simulink model "taskBasedWalking"  (Simulink 8.8)
settings: Solver=FixedStepDiscrete  StartTime=0.0  StopTime=Config.t_end  FixedStep=Config.t_step  RelTol=1e-3  EnableMultiTasking=on
InitFcn:
  | cd(fileparts(which(bdroot)));
  | initTaskBasedWalking;
StopFcn:
  | cd(fileparts(which(bdroot)));
  | stopTaskBasedWalking;
undefined symbols (not defined in the file or in its folder): biasVectorConstraint_feet, Config, ConstraintMatrix_feet, DiscIntNeverNeededParam, Gains, ROBOT_DOF, Sat
libraries: WBToolboxLibrary x78
(part 1 of 3)
settings Model: SuppressorTable=22 serialization::archive 11 0 6 0 0 0 11 0  Creator=gnava  LastModifiedBy=gabri
settings DataIOCC: LimitDataPoints=off  SaveFormat=Dataset  SignalLoggingSaveFormat=Dataset
settings OptimizationCC: LifeSpan=auto
settings DebuggingCC: UnderspecifiedInitializationDetection=Simplified  MergeDetectMultiDrivingBlocksExec=error  FcnCallInpInsideContextMsg=error  StateNameClashWarn=none  SFUnexpectedBacktrackingDiag=error  SFNoUnconditionalDefaultTransitionDiag=error
settings HardwareCC: ProdBitPerPointer=64  ProdBitPerSizeT=64  ProdBitPerPtrDiffT=64  ProdLargestAtomicFloat=Float  ProdIntDivRoundTo=Zero  ProdEndianess=LittleEndian  ProdWordSize=64  ProdHWDeviceType=Intel->x86-64 (Windows64)
settings ModelReferenceCC: PropagateSignalLabelsOutOfModel=on
settings GRTTargetCC: TargetLangStandard=C99 (ISO)  GeneratePreprocessorConditionals=Use local settings  CombineOutputUpdateFcns=on  GRTInterface=off
settings ConfigComp: CovSFcnEnable=off

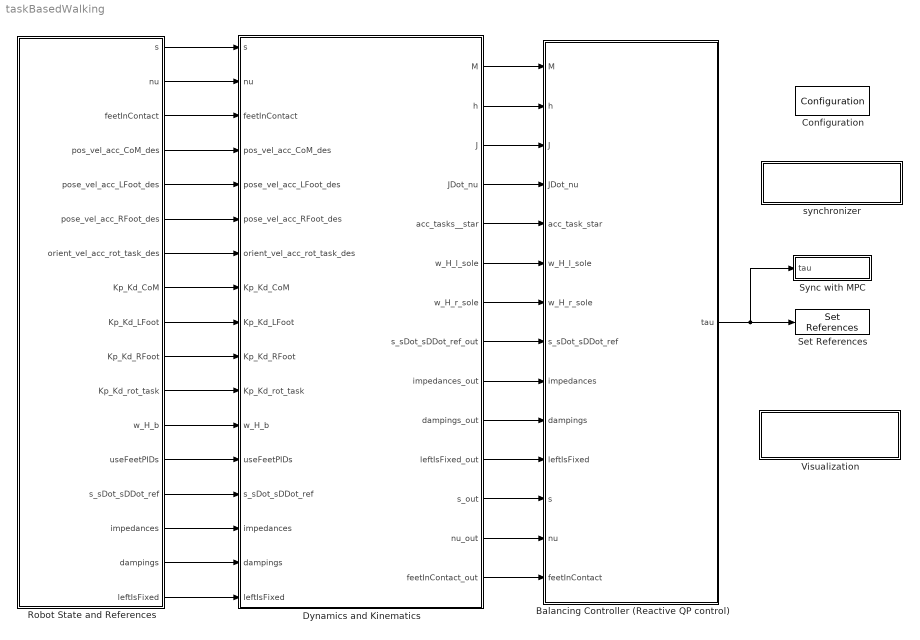
== system taskBasedWalking ==
  Balancing Controller (Reactive QP control) : Subsystem
  Configuration : WBToolboxLibrary/Utilities/Configuration  ConfigSource=Workspace  ConfigObject='WBTConfigRobot'  RobotName='icub'  UrdfFile='model.urdf'  ControlledJoints={'l_elbow','l_shoulder_pitch','torso_roll'}  ControlBoardsNames={'left_arm','right_arm','torso'}  LocalName='WBT'  GravityVector=[0,0,-9.81]
  Dynamics and Kinematics : Subsystem
  Robot State and References : Subsystem
  Set References : WBToolboxLibrary/wholeBodyActuators/Set References  controlType=Torque  refSpeed=50
  Sync with MPC : Subsystem
      mask Display: disp('Sync with MPC')
  Visualization : Subsystem
      mask Display: disp('VISUALIZE AND DUMP DATA')
  synchronizer : Subsystem
      mask Display: disp('SYNCHRONIZER')
  wires:
  Balancing Controller (Reactive QP control)/1(tau) -> Sync with MPC/1(tau), Set References/1
  Robot State and References/1(s) -> Dynamics and Kinematics/1(s)
  Robot State and References/2(nu) -> Dynamics and Kinematics/2(nu)
  Robot State and References/3(feetInContact) -> Dynamics and Kinematics/3(feetInContact)
  Robot State and References/4(pos_vel_acc_CoM_des) -> Dynamics and Kinematics/4(pos_vel_acc_CoM_des)
  Robot State and References/5(pose_vel_acc_LFoot_des) -> Dynamics and Kinematics/5(pose_vel_acc_LFoot_des)
  Robot State and References/6(pose_vel_acc_RFoot_des) -> Dynamics and Kinematics/6(pose_vel_acc_RFoot_des)
  Robot State and References/7(orient_vel_acc_rot_task_des) -> Dynamics and Kinematics/7(orient_vel_acc_rot_task_des)
  Robot State and References/8(Kp_Kd_CoM) -> Dynamics and Kinematics/8(Kp_Kd_CoM)
  Robot State and References/9(Kp_Kd_LFoot) -> Dynamics and Kinematics/9(Kp_Kd_LFoot)
  Robot State and References/10(Kp_Kd_RFoot) -> Dynamics and Kinematics/10(Kp_Kd_RFoot)
  Robot State and References/11(Kp_Kd_rot_task) -> Dynamics and Kinematics/11(Kp_Kd_rot_task)
  Robot State and References/12(w_H_b) -> Dynamics and Kinematics/12(w_H_b)
  Robot State and References/13("useFeetPIDs ") -> Dynamics and Kinematics/13(useFeetPIDs)
  Robot State and References/14(s_sDot_sDDot_ref) -> Dynamics and Kinematics/14(s_sDot_sDDot_ref)
  Robot State and References/15(impedances) -> Dynamics and Kinematics/15(impedances)
  Robot State and References/16(dampings) -> Dynamics and Kinematics/16(dampings)
  Robot State and References/17(leftIsFixed) -> Dynamics and Kinematics/17(leftIsFixed)
  Dynamics and Kinematics/1(M) -> Balancing Controller (Reactive QP control)/1(M)
  Dynamics and Kinematics/2(h) -> Balancing Controller (Reactive QP control)/2(h)
  Dynamics and Kinematics/3(J) -> Balancing Controller (Reactive QP control)/3(J)
  Dynamics and Kinematics/4(JDot_nu) -> Balancing Controller (Reactive QP control)/4(JDot_nu)
  Dynamics and Kinematics/5(acc_tasks__star) -> Balancing Controller (Reactive QP control)/5(acc_task_star)
  Dynamics and Kinematics/6(w_H_l_sole) -> Balancing Controller (Reactive QP control)/6(w_H_l_sole)
  Dynamics and Kinematics/7(w_H_r_sole) -> Balancing Controller (Reactive QP control)/7(w_H_r_sole)
  Dynamics and Kinematics/8(s_sDot_sDDot_ref_out) -> Balancing Controller (Reactive QP control)/8(s_sDot_sDDot_ref)
  Dynamics and Kinematics/9(impedances_out) -> Balancing Controller (Reactive QP control)/9(impedances)
  Dynamics and Kinematics/10(dampings_out) -> Balancing Controller (Reactive QP control)/10(dampings)
  Dynamics and Kinematics/11(leftIsFixed_out) -> Balancing Controller (Reactive QP control)/11(leftIsFixed)
  Dynamics and Kinematics/12(s_out) -> Balancing Controller (Reactive QP control)/12(s)
  Dynamics and Kinematics/13(nu_out) -> Balancing Controller (Reactive QP control)/13(nu)
  Dynamics and Kinematics/14(feetInContact_out) -> Balancing Controller (Reactive QP control)/14(feetInContact)

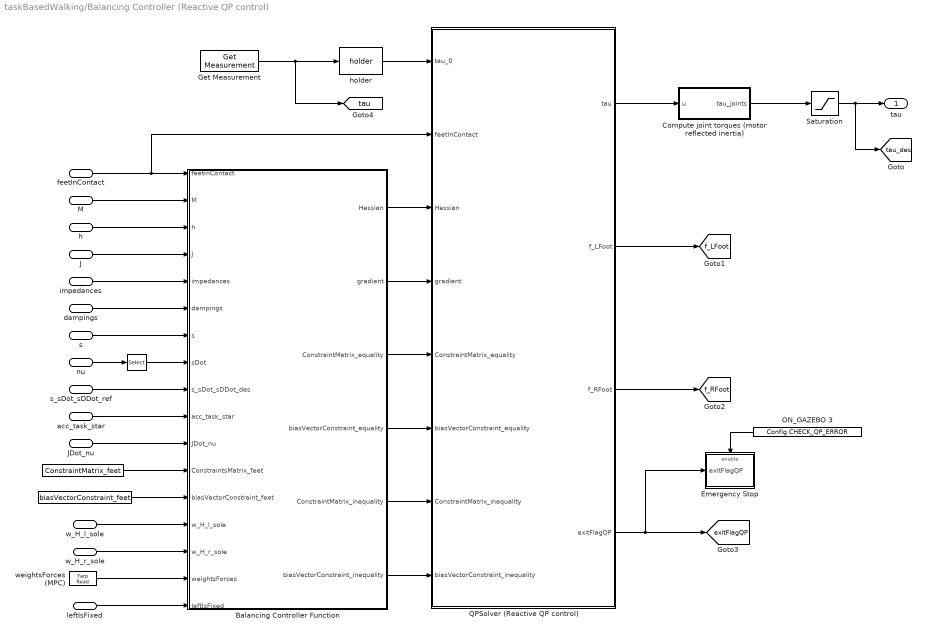
== system taskBasedWalking/Balancing Controller (Reactive QP control) ==
  M : Inport
  h : Inport  Port=2
  J : Inport  Port=3
  JDot_nu : Inport  Port=4
  acc_task_star : Inport  Port=5
  w_H_l_sole : Inport  Port=6
  w_H_r_sole : Inport  Port=7
  s_sDot_sDDot_ref : Inport  Port=8
  impedances : Inport  Port=9
  dampings : Inport  Port=10
  leftIsFixed : Inport  Port=11
  s : Inport  Port=12
  nu : Inport  Port=13
  feetInContact : Inport  Port=14
  "   " : Constant  Value=ConstraintMatrix_feet
  "      " : Constant  Value=biasVectorConstraint_feet
  "             " : Selector  InputPortWidth=ROBOT_DOF+6  IndexOptions=Index vector (dialog)  Indices=[7:ROBOT_DOF+6]  OutputSizes=1
  Balancing Controller Function : MATLAB Function  TreatAsAtomicUnit=on
  Compute joint torques (motor reflected inertia) : Subsystem
  Emergency Stop : Subsystem
  Get Measurement : WBToolboxLibrary/wholeBodyStates/Get Measurement  measuredType=Joints Torque
  ON_GAZEBO 3 : Constant  Value=Config.CHECK_QP_ERROR
  QPSolver (Reactive QP control) : Subsystem
  Saturation : Saturate  UpperLimit=Sat.tau_max  LowerLimit=-Sat.tau_max
  "holder " : WBToolboxLibrary/Utilities/holder 
  weightsForces (MPC) : WBToolboxLibrary/Utilities/Yarp Read  portName=Ports.FORCE_WEIGHTS  signalSize=2  timeout=0.5  blocking=off  timestamp=off  autoconnect=on  errorOnConnection=off
  tau : Outport
  tag scope: exitFlagQP=global, f_LFoot=global, f_RFoot=global, tau=global, tau_des=global
  wires:
  QPSolver (Reactive QP control)/1(tau) -> Compute joint torques (motor reflected inertia)/1(u)
  "holder "/1 -> QPSolver (Reactive QP control)/1(tau_0)
  Balancing Controller Function/3(ConstraintMatrix_equality) -> QPSolver (Reactive QP control)/5(ConstraintMatrix_equality)
  Balancing Controller Function/6(biasVectorConstraint_inequality) -> QPSolver (Reactive QP control)/8(biasVectorConstraint_inequality)
  Balancing Controller Function/2(gradient) -> QPSolver (Reactive QP control)/4(gradient)
  Balancing Controller Function/4(biasVectorConstraint_equality) -> QPSolver (Reactive QP control)/6(biasVectorConstraint_equality)
  Balancing Controller Function/5(ConstraintMatrix_inequality) -> QPSolver (Reactive QP control)/7(ConstraintMatrix_inequality)
  w_H_r_sole/1 -> Balancing Controller Function/15(w_H_r_sole)
  w_H_l_sole/1 -> Balancing Controller Function/14(w_H_l_sole)
  "      "/1 -> Balancing Controller Function/13(biasVectorConstraint_feet)
  "   "/1 -> Balancing Controller Function/12(ConstraintsMatrix_feet)
  JDot_nu/1 -> Balancing Controller Function/11(JDot_nu)
  acc_task_star/1 -> Balancing Controller Function/10(acc_task_star)
  s_sDot_sDDot_ref/1 -> Balancing Controller Function/9(s_sDot_sDDot_des)
  nu/1 -> "             "/1
  s/1 -> Balancing Controller Function/7(s)
  dampings/1 -> Balancing Controller Function/6(dampings)
  impedances/1 -> Balancing Controller Function/5(impedances)
  J/1 -> Balancing Controller Function/4(J)
  h/1 -> Balancing Controller Function/3(h)
  M/1 -> Balancing Controller Function/2(M)
  Get Measurement/1 -> [tau], "holder "/1
  "             "/1 -> Balancing Controller Function/8(sDot)
  Saturation/1 -> tau/1, [tau_des]
  Balancing Controller Function/1(Hessian) -> QPSolver (Reactive QP control)/3(Hessian)
  feetInContact/1 -> Balancing Controller Function/1(feetInContact), QPSolver (Reactive QP control)/2(feetInContact)
  QPSolver (Reactive QP control)/2(f_LFoot) -> [f_LFoot]
  QPSolver (Reactive QP control)/3(f_RFoot) -> [f_RFoot]
  QPSolver (Reactive QP control)/4(exitFlagQP) -> Emergency Stop/1(exitFlagQP), [exitFlagQP]
  ON_GAZEBO 3/1 -> Emergency Stop/Enable
  Compute joint torques (motor reflected inertia)/1(tau_joints) -> Saturation/1
  weightsForces (MPC)/1 -> Balancing Controller Function/16(weightsForces)
  leftIsFixed/1 -> Balancing Controller Function/17(leftIsFixed)

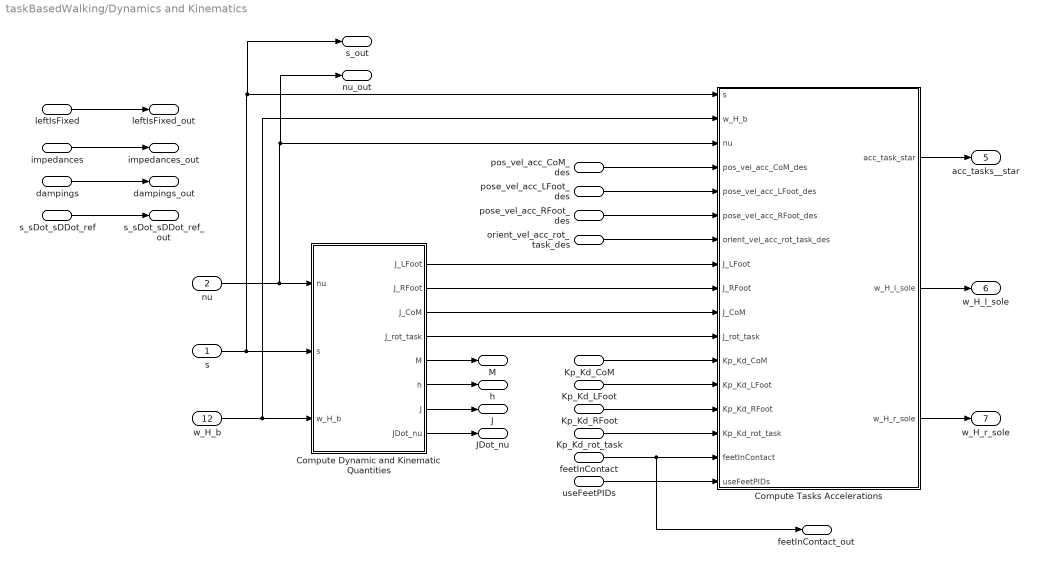
== system taskBasedWalking/Dynamics and Kinematics ==
  s : Inport
  nu : Inport  Port=2
  feetInContact : Inport  Port=3
  pos_vel_acc_CoM_des : Inport  Port=4
  pose_vel_acc_LFoot_des : Inport  Port=5
  pose_vel_acc_RFoot_des : Inport  Port=6
  orient_vel_acc_rot_task_des : Inport  Port=7
  Kp_Kd_CoM : Inport  Port=8
  Kp_Kd_LFoot : Inport  Port=9
  Kp_Kd_RFoot : Inport  Port=10
  Kp_Kd_rot_task : Inport  Port=11
  w_H_b : Inport  Port=12
  useFeetPIDs : Inport  Port=13
  s_sDot_sDDot_ref : Inport  Port=14
  impedances : Inport  Port=15
  dampings : Inport  Port=16
  leftIsFixed : Inport  Port=17
  Compute Dynamic and Kinematic Quantities : Subsystem
  Compute Tasks Accelerations : Subsystem
  M : Outport
  h : Outport  Port=2
  J : Outport  Port=3
  JDot_nu : Outport  Port=4
  acc_tasks__star : Outport  Port=5
  w_H_l_sole : Outport  Port=6
  w_H_r_sole : Outport  Port=7
  s_sDot_sDDot_ref_out : Outport  Port=8
  impedances_out : Outport  Port=9
  dampings_out : Outport  Port=10
  leftIsFixed_out : Outport  Port=11
  s_out : Outport  Port=12
  nu_out : Outport  Port=13
  feetInContact_out : Outport  Port=14
  wires:
  pos_vel_acc_CoM_des/1 -> Compute Tasks Accelerations/4(pos_vel_acc_CoM_des)
  pose_vel_acc_LFoot_des/1 -> Compute Tasks Accelerations/5(pose_vel_acc_LFoot_des)
  pose_vel_acc_RFoot_des/1 -> Compute Tasks Accelerations/6(pose_vel_acc_RFoot_des)
  orient_vel_acc_rot_task_des/1 -> Compute Tasks Accelerations/7(orient_vel_acc_rot_task_des)
  Kp_Kd_CoM/1 -> Compute Tasks Accelerations/12(Kp_Kd_CoM)
  Kp_Kd_LFoot/1 -> Compute Tasks Accelerations/13(Kp_Kd_LFoot)
  Kp_Kd_RFoot/1 -> Compute Tasks Accelerations/14(Kp_Kd_RFoot)
  Kp_Kd_rot_task/1 -> Compute Tasks Accelerations/15(Kp_Kd_rot_task)
  nu/1 -> Compute Dynamic and Kinematic Quantities/1(nu), nu_out/1, Compute Tasks Accelerations/3(nu)
  s/1 -> Compute Dynamic and Kinematic Quantities/2(s), s_out/1, Compute Tasks Accelerations/1(s)
  w_H_b/1 -> Compute Dynamic and Kinematic Quantities/3(w_H_b), Compute Tasks Accelerations/2(w_H_b)
  Compute Dynamic and Kinematic Quantities/6(h) -> h/1
  Compute Dynamic and Kinematic Quantities/1(J_LFoot) -> Compute Tasks Accelerations/8(J_LFoot)
  Compute Dynamic and Kinematic Quantities/2(J_RFoot) -> Compute Tasks Accelerations/9(J_RFoot)
  Compute Dynamic and Kinematic Quantities/3(J_CoM) -> Compute Tasks Accelerations/10(J_CoM)
  Compute Dynamic and Kinematic Quantities/5(M) -> M/1
  Compute Dynamic and Kinematic Quantities/4(J_rot_task) -> Compute Tasks Accelerations/11(J_rot_task)
  Compute Dynamic and Kinematic Quantities/7(J) -> J/1
  Compute Dynamic and Kinematic Quantities/8(JDot_nu) -> JDot_nu/1
  Compute Tasks Accelerations/2(w_H_l_sole) -> w_H_l_sole/1
  Compute Tasks Accelerations/3(w_H_r_sole) -> w_H_r_sole/1
  Compute Tasks Accelerations/1(acc_task_star) -> acc_tasks__star/1
  useFeetPIDs/1 -> Compute Tasks Accelerations/17(useFeetPIDs)
  leftIsFixed/1 -> leftIsFixed_out/1
  impedances/1 -> impedances_out/1
  dampings/1 -> dampings_out/1
  s_sDot_sDDot_ref/1 -> s_sDot_sDDot_ref_out/1
  feetInContact/1 -> feetInContact_out/1, Compute Tasks Accelerations/16(feetInContact)

== system taskBasedWalking/Robot State and References ==
  Gain Scheduling : Subsystem
  ON_GAZEBO 1 : Constant  Value=Config.CHECK_LIMITS
  "Smooth References " : Subsystem
  State Machine : Subsystem
  emergency stop: joint limits : Subsystem
  s : Outport
  nu : Outport  Port=2
  feetInContact : Outport  Port=3
  pos_vel_acc_CoM_des : Outport  Port=4
  pose_vel_acc_LFoot_des : Outport  Port=5
  pose_vel_acc_RFoot_des : Outport  Port=6
  orient_vel_acc_rot_task_des : Outport  Port=7
  Kp_Kd_CoM : Outport  Port=8
  Kp_Kd_LFoot : Outport  Port=9
  Kp_Kd_RFoot : Outport  Port=10
  Kp_Kd_rot_task : Outport  Port=11
  w_H_b : Outport  Port=12
  "useFeetPIDs " : Outport  Port=13
  s_sDot_sDDot_ref : Outport  Port=14
  impedances : Outport  Port=15
  dampings : Outport  Port=16
  leftIsFixed : Outport  Port=17
  wires:
  Gain Scheduling/1(Kp_Kd_CoM) -> Kp_Kd_CoM/1
  Gain Scheduling/2(Kp_Kd_LFoot) -> Kp_Kd_LFoot/1
  Gain Scheduling/3(Kp_Kd_RFoot) -> Kp_Kd_RFoot/1
  Gain Scheduling/4(Kp_Kd_rot_task) -> Kp_Kd_rot_task/1
  Gain Scheduling/5(impedances) -> impedances/1
  Gain Scheduling/6(dampings) -> dampings/1
  "Smooth References "/1(pos_vel_acc_CoM_des) -> pos_vel_acc_CoM_des/1
  "Smooth References "/2(pose_vel_acc_LFoot_des) -> pose_vel_acc_LFoot_des/1
  "Smooth References "/3(pose_vel_acc_RFoot_des) -> pose_vel_acc_RFoot_des/1
  "Smooth References "/4(orient_vel_acc_rot_task_des) -> orient_vel_acc_rot_task_des/1
  "Smooth References "/5(s_sDot_sDDot_ref) -> s_sDot_sDDot_ref/1
  ON_GAZEBO 1/1 -> emergency stop: joint limits/Enable
  State Machine/1(s) -> s/1, emergency stop: joint limits/1(s   EMERGENCY STOP)
  State Machine/2(w_H_b) -> w_H_b/1
  State Machine/3(nu) -> nu/1
  State Machine/4(feetInContact) -> feetInContact/1
  State Machine/5(leftIsFixed) -> leftIsFixed/1
  State Machine/7(state) -> "Smooth References "/1(state), Gain Scheduling/1(state)
  State Machine/8(references_CoM) -> "Smooth References "/2(references_CoM)
  State Machine/9(references_LFoot) -> "Smooth References "/3(references_LFoot)
  State Machine/10(references_RFoot) -> "Smooth References "/4(references_RFoot)
  State Machine/11(references_rot_task) -> "Smooth References "/5(references_rot_task)
  State Machine/12(references_s) -> "Smooth References "/6(references_s)
  State Machine/6(useFeetPIDs) -> "useFeetPIDs "/1

== system taskBasedWalking/Sync with MPC ==
  tau : Inport
  Clock : Clock
  Gain : Gain  Gain=0
  Mux : Mux  Inputs=2
  Selector : Selector  InputPortWidth=ROBOT_DOF  IndexOptions=Index vector (dialog)  Indices=[1]  OutputSizes=1
  Yarp Write : WBToolboxLibrary/Utilities/Yarp Write  portName=Ports.ACK  autoconnect=on  errorOnConnection=off
  wires:
  Clock/1 -> Mux/2
  tau/1 -> Selector/1
  Mux/1 -> Yarp Write/1
  Selector/1 -> Gain/1
  Gain/1 -> Mux/1

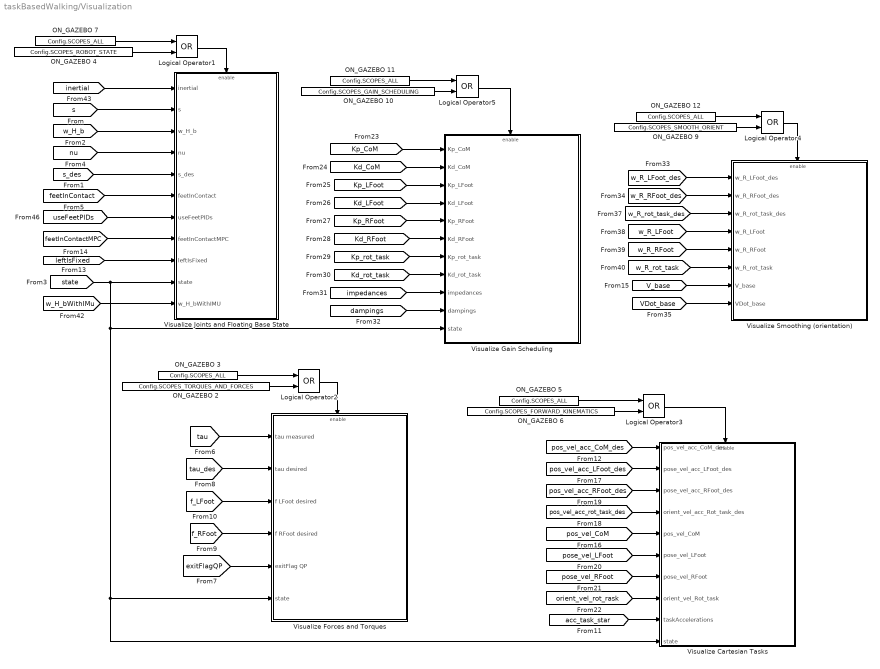
== system taskBasedWalking/Visualization ==
  Logical Operator{1..5} (5 alike) : Logic  Operator=OR  AllPortsSameDT=off  OutDataTypeStr=boolean
  ON_GAZEBO 10 : Constant  Value=Config.SCOPES_GAIN_SCHEDULING
  ON_GAZEBO {3,5,7,11..12} (5 alike) : Constant  Value=Config.SCOPES_ALL
  ON_GAZEBO 2 : Constant  Value=Config.SCOPES_TORQUES_AND_FORCES
  ON_GAZEBO 4 : Constant  Value=Config.SCOPES_ROBOT_STATE
  ON_GAZEBO 6 : Constant  Value=Config.SCOPES_FORWARD_KINEMATICS
  ON_GAZEBO 9 : Constant  Value=Config.SCOPES_SMOOTH_ORIENT
  Visualize Cartesian Tasks : Subsystem
  Visualize Forces and Torques : Subsystem
  Visualize Gain Scheduling : Subsystem
  Visualize Joints and Floating Base State : Subsystem
  Visualize Smoothing (orientation) : Subsystem
  wires:
  [s] -> Visualize Joints and Floating Base State/2(s)
  [w_H_b] -> Visualize Joints and Floating Base State/3(w_H_b)
  [s_des] -> Visualize Joints and Floating Base State/5(s_des)
  [nu] -> Visualize Joints and Floating Base State/4(nu)
  [state] -> Visualize Cartesian Tasks/10(state), Visualize Forces and Torques/6(state), Visualize Gain Scheduling/11(state), Visualize Joints and Floating Base State/10(state)
  [tau] -> Visualize Forces and Torques/1(tau measured)
  [tau_des] -> Visualize Forces and Torques/2(tau desired)
  [f_LFoot] -> Visualize Forces and Torques/3(f LFoot desired)
  [f_RFoot] -> Visualize Forces and Torques/4(f RFoot desired)
  [exitFlagQP] -> Visualize Forces and Torques/5(exitFlag QP)
  ON_GAZEBO 4/1 -> Logical Operator1/2
  ON_GAZEBO 7/1 -> Logical Operator1/1
  Logical Operator1/1 -> Visualize Joints and Floating Base State/Enable
  [feetInContact] -> Visualize Joints and Floating Base State/6(feetInContact)
  Logical Operator2/1 -> Visualize Forces and Torques/Enable
  ON_GAZEBO 3/1 -> Logical Operator2/1
  ON_GAZEBO 2/1 -> Logical Operator2/2
  ON_GAZEBO 6/1 -> Logical Operator3/2
  Logical Operator3/1 -> Visualize Cartesian Tasks/Enable
  ON_GAZEBO 5/1 -> Logical Operator3/1
  [pos_vel_acc_CoM_des] -> Visualize Cartesian Tasks/1(pos_vel_acc_CoM_des)
  [pos_vel_acc_LFoot_des] -> Visualize Cartesian Tasks/2(pose_vel_acc_LFoot_des)
  [pos_vel_acc_RFoot_des] -> Visualize Cartesian Tasks/3(pose_vel_acc_RFoot_des)
  [pos_vel_acc_rot_task_des] -> Visualize Cartesian Tasks/4(orient_vel_acc_Rot_task_des)
  [pos_vel_CoM] -> Visualize Cartesian Tasks/5(pos_vel_CoM)
  [pose_vel_LFoot] -> Visualize Cartesian Tasks/6(pose_vel_LFoot)
  [pose_vel_RFoot] -> Visualize Cartesian Tasks/7(pose_vel_RFoot)
  [orient_vel_rot_rask] -> Visualize Cartesian Tasks/8(orient_vel_Rot_task)
  ON_GAZEBO 10/1 -> Logical Operator5/2
  ON_GAZEBO 11/1 -> Logical Operator5/1
  Logical Operator5/1 -> Visualize Gain Scheduling/Enable
  [Kp_CoM] -> Visualize Gain Scheduling/1(Kp_CoM)
  [Kd_CoM] -> Visualize Gain Scheduling/2(Kd_CoM)
  [Kp_LFoot] -> Visualize Gain Scheduling/3(Kp_LFoot)
  [Kd_LFoot] -> Visualize Gain Scheduling/4(Kd_LFoot)
  [Kp_RFoot] -> Visualize Gain Scheduling/5(Kp_RFoot)
  [Kd_RFoot] -> Visualize Gain Scheduling/6(Kd_RFoot)
  [Kp_rot_task] -> Visualize Gain Scheduling/7(Kp_rot_task)
  [Kd_rot_task] -> Visualize Gain Scheduling/8(Kd_rot_task)
  [impedances] -> Visualize Gain Scheduling/9(impedances)
  [dampings] -> Visualize Gain Scheduling/10(dampings)
  ON_GAZEBO 9/1 -> Logical Operator4/2
  ON_GAZEBO 12/1 -> Logical Operator4/1
  Logical Operator4/1 -> Visualize Smoothing (orientation)/Enable
  [w_R_LFoot_des] -> Visualize Smoothing (orientation)/1(w_R_LFoot_des)
  [w_R_RFoot_des] -> Visualize Smoothing (orientation)/2(w_R_RFoot_des)
  [w_R_rot_task_des] -> Visualize Smoothing (orientation)/3(w_R_rot_task_des)
  [w_R_LFoot] -> Visualize Smoothing (orientation)/4(w_R_LFoot)
  [w_R_RFoot] -> Visualize Smoothing (orientation)/5(w_R_RFoot)
  [w_R_rot_task] -> Visualize Smoothing (orientation)/6(w_R_rot_task)
  [acc_task_star] -> Visualize Cartesian Tasks/9(taskAccelerations)
  [leftIsFixed] -> Visualize Joints and Floating Base State/9(leftIsFixed)
  [useFeetPIDs] -> Visualize Joints and Floating Base State/7(useFeetPIDs)
  [feetInContactMPC] -> Visualize Joints and Floating Base State/8(feetInContactMPC)
  [V_base] -> Visualize Smoothing (orientation)/7(V_base)
  [VDot_base] -> Visualize Smoothing (orientation)/8(VDot_base)
  [w_H_bWithIMu] -> Visualize Joints and Floating Base State/11(w_H_bWithIMU)
  [inertial] -> Visualize Joints and Floating Base State/1(inertial)

== system taskBasedWalking/synchronizer ==
  GAZEBO_SYNCHRONIZER : Subsystem
  Logical Operator : Logic  Operator=NOT  AllPortsSameDT=off  OutDataTypeStr=boolean
  "ON_GAZEBO " : Constant  Value=Config.ON_GAZEBO
  REAL_TIME_SYNC : Subsystem
  wires:
  Logical Operator/1 -> REAL_TIME_SYNC/Enable
  "ON_GAZEBO "/1 -> Logical Operator/1, GAZEBO_SYNCHRONIZER/Enable

== system taskBasedWalking/Balancing Controller (Reactive QP control)/Compute joint torques (motor reflected inertia) ==
  u : Inport
  " " : Constant  Value=Config.USE_MOTOR_REFLECTED_INERTIA
  "(transpose(T*Gamma))^{-1}*I_m*(T*Gamma)^{-1}" : MATLAB Function  TreatAsAtomicUnit=on
  Add : Sum  Inputs=-+
  DoFs converter1 : WBToolboxLibrary/Utilities/DoFs converter  yarp2WBIOption=From YARP to WBI
  DoFs converter2 : WBToolboxLibrary/Utilities/DoFs converter  yarp2WBIOption=From YARP to WBI
  Gain : Gain  Gain=Config.K_ff
  Get Measurement : WBToolboxLibrary/wholeBodyStates/Get Measurement  measuredType=Joints Acceleration
  Product : Product  Multiplication=Matrix(*)
  Switch : Switch  Criteria=u2 > Threshold
  joint accelerations : Scope  NumInputPorts=6
  motor reflected inertia ff terms : Scope  NumInputPorts=6
  tau_joints : Outport
  wires:
  Gain/1 -> Add/1
  Add/1 -> Switch/1
  " "/1 -> Switch/2
  Switch/1 -> tau_joints/1
  u/1 -> Add/2, Switch/3
  "(transpose(T*Gamma))^{-1}*I_m*(T*Gamma)^{-1}"/1(reflectedInertia) -> Product/1
  Get Measurement/1 -> DoFs converter1/1, Product/2
  DoFs converter1/4 -> joint accelerations/4  "left_leg"
  DoFs converter1/3 -> joint accelerations/3  "right_arm"
  DoFs converter1/5 -> joint accelerations/5  "right_leg"
  DoFs converter1/2 -> joint accelerations/2  "left_arm"
  DoFs converter1/1 -> joint accelerations/1  "torso"
  DoFs converter2/1 -> motor reflected inertia ff terms/1  "torso"
  DoFs converter2/3 -> motor reflected inertia ff terms/3  "right_arm"
  DoFs converter2/2 -> motor reflected inertia ff terms/2  "left_arm"
  DoFs converter2/5 -> motor reflected inertia ff terms/5  "right_leg"
  Product/1 -> DoFs converter2/1, Gain/1
  DoFs converter2/4 -> motor reflected inertia ff terms/4  "left_leg"

== system taskBasedWalking/Balancing Controller (Reactive QP control)/Emergency Stop ==
  exitFlagQP : Inport
  Enable : EnablePort
  Constant : Constant  Value=2
  Constant1 : Constant  Value=0  OutDataTypeStr=boolean
  Constant2 : Constant  OutDataTypeStr=boolean
  Stop Simulation : Stop
  Sum : Sum  Inputs=|++
  Switch : Switch  Criteria=u2 > Threshold  Threshold=0.1
  wires:
  exitFlagQP/1 -> Sum/1
  Sum/1 -> Switch/2
  Switch/1 -> Stop Simulation/1
  Constant/1 -> Sum/2
  Constant1/1 -> Switch/1
  Constant2/1 -> Switch/3

== system taskBasedWalking/Balancing Controller (Reactive QP control)/QPSolver (Reactive QP control) ==
  tau_0 : Inport
  feetInContact : Inport  Port=2
  Hessian : Inport  Port=3
  gradient : Inport  Port=4
  ConstraintMatrix_equality : Inport  Port=5
  biasVectorConstraint_equality : Inport  Port=6
  ConstraintMatrix_inequality : Inport  Port=7
  biasVectorConstraint_inequality : Inport  Port=8
  QPSolver : M-S-Function  FunctionName=QPBalancingMPC  Parameters=ROBOT_DOF, Sat, Config
  tau : Outport
  f_LFoot : Outport  Port=2
  f_RFoot : Outport  Port=3
  exitFlagQP : Outport  Port=4
  wires:
  gradient/1 -> QPSolver/4
  Hessian/1 -> QPSolver/3
  biasVectorConstraint_inequality/1 -> QPSolver/8
  feetInContact/1 -> QPSolver/2
  QPSolver/2 -> f_LFoot/1
  ConstraintMatrix_inequality/1 -> QPSolver/7
  biasVectorConstraint_equality/1 -> QPSolver/6
  ConstraintMatrix_equality/1 -> QPSolver/5
  tau_0/1 -> QPSolver/1
  QPSolver/1 -> tau/1
  QPSolver/3 -> f_RFoot/1
  QPSolver/4 -> exitFlagQP/1

== system taskBasedWalking/Dynamics and Kinematics/Compute Dynamic and Kinematic Quantities ==
  nu : Inport
  s : Inport  Port=2
  w_H_b : Inport  Port=3
  "  " : Selector  NumberOfDimensions=2  InputPortWidth=ROBOT_DOF+16  IndexOptions=Index vector (dialog),Index vector (dialog)  Indices=[1:3],[1:ROBOT_DOF+6]  OutputSizes=1,1
  "   " : Selector  InputPortWidth=6  IndexOptions=Index vector (dialog)  Indices=[1:3]  OutputSizes=1
  "     " : Selector  NumberOfDimensions=2  InputPortWidth=ROBOT_DOF+16  IndexOptions=Index vector (dialog),Index vector (dialog)  Indices=[4:6],[1:ROBOT_DOF+6]  OutputSizes=1,1
  "               " : Selector  InputPortWidth=6  IndexOptions=Index vector (dialog)  Indices=[4:6]  OutputSizes=1
  Jacobians and JDot_nu : Subsystem
  Mass Matrix and Bias Forces : Subsystem
  Matrix Concatenate : Concatenate  NumInputs=4  Mode=Multidimensional array
  Selector : Selector  InputPortWidth=ROBOT_DOF+6  IndexOptions=Index vector (dialog)  Indices=[1:6]  OutputSizes=1
  Selector1 : Selector  InputPortWidth=ROBOT_DOF+6  IndexOptions=Index vector (dialog)  Indices=[7:ROBOT_DOF+6]  OutputSizes=1
  Vector Concatenate : Concatenate  NumInputs=4
  J_LFoot : Outport
  J_RFoot : Outport  Port=2
  J_CoM : Outport  Port=3
  J_rot_task : Outport  Port=4
  M : Outport  Port=5
  h : Outport  Port=6
  J : Outport  Port=7
  JDot_nu : Outport  Port=8
  wires:
  "               "/1 -> Vector Concatenate/4
  "  "/1 -> J_CoM/1, Matrix Concatenate/3
  "     "/1 -> J_rot_task/1, Matrix Concatenate/4
  Vector Concatenate/1 -> JDot_nu/1
  Selector1/1 -> Mass Matrix and Bias Forces/3(sDot), Jacobians and JDot_nu/3(sDot)
  Matrix Concatenate/1 -> J/1
  nu/1 -> Selector/1, Selector1/1
  Selector/1 -> Mass Matrix and Bias Forces/2(nu_b), Jacobians and JDot_nu/2(nu_b)
  "   "/1 -> Vector Concatenate/3
  Mass Matrix and Bias Forces/2(M(q)) -> M/1
  Mass Matrix and Bias Forces/1(h(q,nu)) -> h/1
  s/1 -> Jacobians and JDot_nu/1(s), Mass Matrix and Bias Forces/1(s)
  w_H_b/1 -> Jacobians and JDot_nu/4(w_H_b), Mass Matrix and Bias Forces/4(w_H_b)
  Jacobians and JDot_nu/2(J_RFoot) -> J_RFoot/1, Matrix Concatenate/2
  Jacobians and JDot_nu/1(J_LFoot) -> J_LFoot/1, Matrix Concatenate/1
  Jacobians and JDot_nu/3(J_CoM) -> "  "/1
  Jacobians and JDot_nu/4(J_rot_task) -> "     "/1
  Jacobians and JDot_nu/5(JDot_nu_LFoot) -> Vector Concatenate/1
  Jacobians and JDot_nu/6(JDot_nu_RFoot) -> Vector Concatenate/2
  Jacobians and JDot_nu/7(JDot_nu_CoM) -> "   "/1
  Jacobians and JDot_nu/8(JDot_nu_rot_task) -> "               "/1

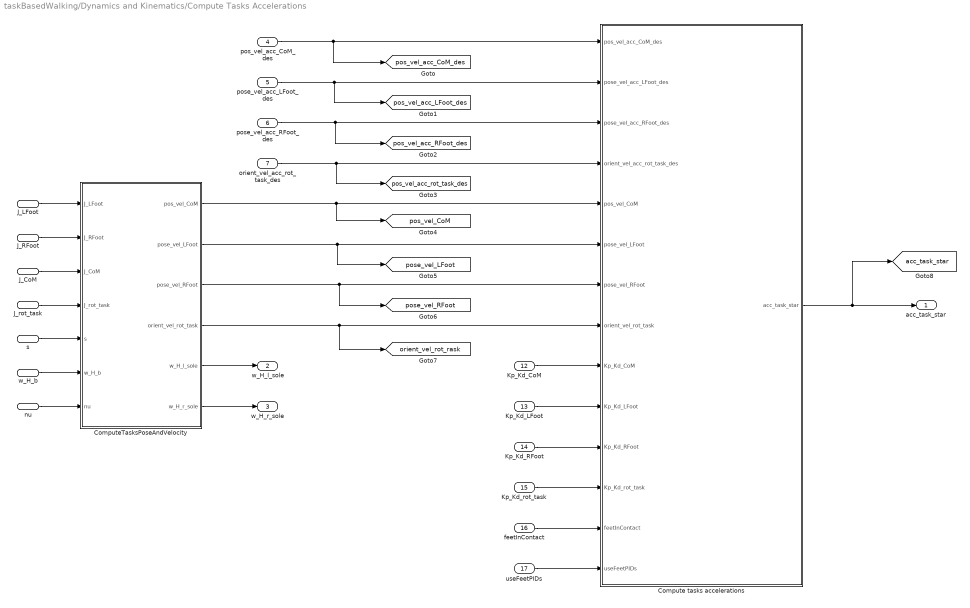
== system taskBasedWalking/Dynamics and Kinematics/Compute Tasks Accelerations ==
  s : Inport
  w_H_b : Inport  Port=2
  nu : Inport  Port=3
  pos_vel_acc_CoM_des : Inport  Port=4
  pose_vel_acc_LFoot_des : Inport  Port=5
  pose_vel_acc_RFoot_des : Inport  Port=6
  orient_vel_acc_rot_task_des : Inport  Port=7
  J_LFoot : Inport  Port=8
  J_RFoot : Inport  Port=9
  J_CoM : Inport  Port=10
  J_rot_task : Inport  Port=11
  Kp_Kd_CoM : Inport  Port=12
  Kp_Kd_LFoot : Inport  Port=13
  Kp_Kd_RFoot : Inport  Port=14
  Kp_Kd_rot_task : Inport  Port=15
  feetInContact : Inport  Port=16
  useFeetPIDs : Inport  Port=17
  Compute tasks accelerations : MATLAB Function  TreatAsAtomicUnit=on
  ComputeTasksPoseAndVelocity : Subsystem
  acc_task_star : Outport
  w_H_l_sole : Outport  Port=2
  w_H_r_sole : Outport  Port=3
  tag scope: acc_task_star=global, orient_vel_rot_rask=global, pos_vel_CoM=global, pos_vel_acc_CoM_des=global, pos_vel_acc_LFoot_des=global, pos_vel_acc_RFoot_des=global, pos_vel_acc_rot_task_des=global, pose_vel_LFoot=global, pose_vel_RFoot=global
  wires:
  pos_vel_acc_CoM_des/1 -> Compute tasks accelerations/1(pos_vel_acc_CoM_des), [pos_vel_acc_CoM_des]
  Kp_Kd_RFoot/1 -> Compute tasks accelerations/11(Kp_Kd_RFoot)
  Kp_Kd_rot_task/1 -> Compute tasks accelerations/12(Kp_Kd_rot_task)
  feetInContact/1 -> Compute tasks accelerations/13(feetInContact)
  pose_vel_acc_RFoot_des/1 -> [pos_vel_acc_RFoot_des], Compute tasks accelerations/3(pose_vel_acc_RFoot_des)
  Kp_Kd_LFoot/1 -> Compute tasks accelerations/10(Kp_Kd_LFoot)
  Kp_Kd_CoM/1 -> Compute tasks accelerations/9(Kp_Kd_CoM)
  orient_vel_acc_rot_task_des/1 -> [pos_vel_acc_rot_task_des], Compute tasks accelerations/4(orient_vel_acc_rot_task_des)
  pose_vel_acc_LFoot_des/1 -> [pos_vel_acc_LFoot_des], Compute tasks accelerations/2(pose_vel_acc_LFoot_des)
  Compute tasks accelerations/1(acc_task_star) -> [acc_task_star], acc_task_star/1
  ComputeTasksPoseAndVelocity/1(pos_vel_CoM) -> [pos_vel_CoM], Compute tasks accelerations/5(pos_vel_CoM)
  ComputeTasksPoseAndVelocity/4(orient_vel_rot_task) -> [orient_vel_rot_rask], Compute tasks accelerations/8(orient_vel_rot_task)
  J_LFoot/1 -> ComputeTasksPoseAndVelocity/1(J_LFoot)
  J_RFoot/1 -> ComputeTasksPoseAndVelocity/2(J_RFoot)
  J_CoM/1 -> ComputeTasksPoseAndVelocity/3(J_CoM)
  J_rot_task/1 -> ComputeTasksPoseAndVelocity/4(J_rot_task)
  s/1 -> ComputeTasksPoseAndVelocity/5(s)
  w_H_b/1 -> ComputeTasksPoseAndVelocity/6(w_H_b)
  nu/1 -> ComputeTasksPoseAndVelocity/7(nu)
  ComputeTasksPoseAndVelocity/2(pose_vel_LFoot) -> [pose_vel_LFoot], Compute tasks accelerations/6(pose_vel_LFoot)
  ComputeTasksPoseAndVelocity/3(pose_vel_RFoot) -> [pose_vel_RFoot], Compute tasks accelerations/7(pose_vel_RFoot)
  ComputeTasksPoseAndVelocity/5(w_H_l_sole) -> w_H_l_sole/1
  ComputeTasksPoseAndVelocity/6(w_H_r_sole) -> w_H_r_sole/1
  useFeetPIDs/1 -> Compute tasks accelerations/14(useFeetPIDs)

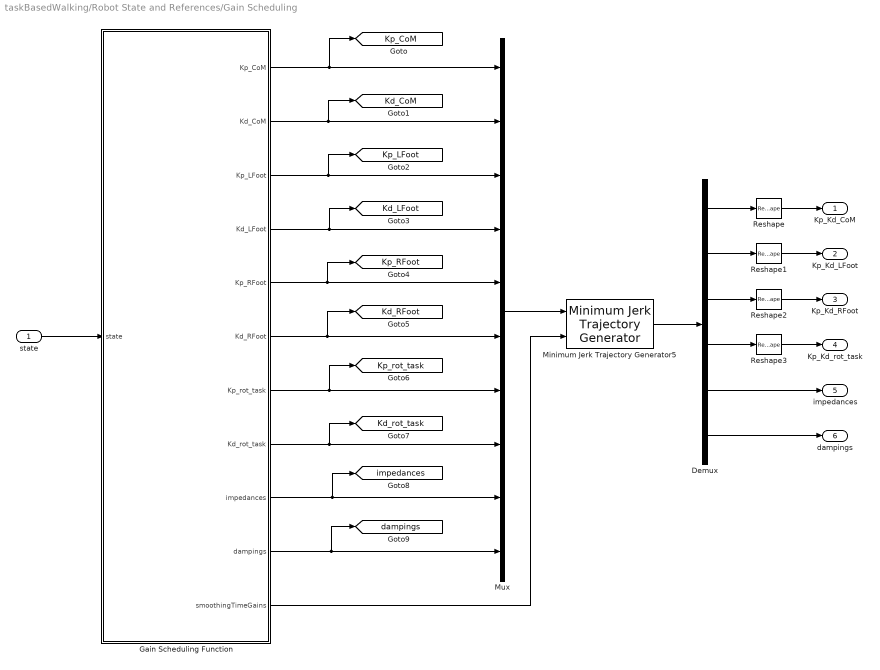
== system taskBasedWalking/Robot State and References/Gain Scheduling ==
  state : Inport
  Demux : Demux  Outputs=[6;12;12;6;ROBOT_DOF;ROBOT_DOF]
  Gain Scheduling Function : MATLAB Function  TreatAsAtomicUnit=on
  Minimum Jerk Trajectory Generator5 : WBToolboxLibrary/Utilities/Minimum Jerk Trajectory Generator  externalSettlingTime=on  settlingTime=3  sampleTime=Config.t_step  resetOnSettlingTime=off  firstDerivatives=off  secondDerivatives=off  explicitInitialValue=off
  Mux : Mux  Inputs=10
  Reshape : Reshape  OutputDimensionality=Customize  OutputDimensions=[3;2]
  Reshape1 : Reshape  OutputDimensionality=Customize  OutputDimensions=[6;2]
  Reshape2 : Reshape  OutputDimensionality=Customize  OutputDimensions=[6;2]
  Reshape3 : Reshape  OutputDimensionality=Customize  OutputDimensions=[3;2]
  Kp_Kd_CoM : Outport
  Kp_Kd_LFoot : Outport  Port=2
  Kp_Kd_RFoot : Outport  Port=3
  Kp_Kd_rot_task : Outport  Port=4
  impedances : Outport  Port=5
  dampings : Outport  Port=6
  tag scope: Kd_CoM=global, Kd_LFoot=global, Kd_RFoot=global, Kd_rot_task=global, Kp_CoM=global, Kp_LFoot=global, Kp_RFoot=global, Kp_rot_task=global, dampings=global, impedances=global
  wires:
  state/1 -> Gain Scheduling Function/1(state)
  Gain Scheduling Function/1(Kp_CoM) -> [Kp_CoM], Mux/1
  Gain Scheduling Function/2(Kd_CoM) -> [Kd_CoM], Mux/2
  Gain Scheduling Function/3(Kp_LFoot) -> [Kp_LFoot], Mux/3
  Gain Scheduling Function/4(Kd_LFoot) -> [Kd_LFoot], Mux/4
  Gain Scheduling Function/5(Kp_RFoot) -> [Kp_RFoot], Mux/5
  Gain Scheduling Function/6(Kd_RFoot) -> [Kd_RFoot], Mux/6
  Gain Scheduling Function/7(Kp_rot_task) -> [Kp_rot_task], Mux/7
  Gain Scheduling Function/8(Kd_rot_task) -> [Kd_rot_task], Mux/8
  Mux/1 -> Minimum Jerk Trajectory Generator5/1
  Gain Scheduling Function/9(impedances) -> [impedances], Mux/9
  Gain Scheduling Function/10(dampings) -> [dampings], Mux/10
  Gain Scheduling Function/11(smoothingTimeGains) -> Minimum Jerk Trajectory Generator5/2
  Minimum Jerk Trajectory Generator5/1 -> Demux/1
  Demux/1 -> Reshape/1
  Demux/2 -> Reshape1/1
  Demux/3 -> Reshape2/1
  Demux/4 -> Reshape3/1
  Reshape/1 -> Kp_Kd_CoM/1
  Reshape1/1 -> Kp_Kd_LFoot/1
  Reshape2/1 -> Kp_Kd_RFoot/1
  Reshape3/1 -> Kp_Kd_rot_task/1
  Demux/5 -> impedances/1
  Demux/6 -> dampings/1

== system taskBasedWalking/Robot State and References/Smooth References  ==
  state : Inport
  references_CoM : Inport  Port=2
  references_LFoot : Inport  Port=3
  references_RFoot : Inport  Port=4
  references_rot_task : Inport  Port=5
  references_s : Inport  Port=6
  Choose Smoothed or Direct References : Subsystem
  Selector1 : Selector  NumberOfDimensions=2  InputPortWidth=3  IndexOptions=Index vector (dialog),Index vector (dialog)  Indices=[1:3],1  OutputSizes=1,1
  Selector2 : Selector  NumberOfDimensions=2  InputPortWidth=3  IndexOptions=Index vector (dialog),Index vector (dialog)  Indices=[1:3],1  OutputSizes=1,1
  Selector3 : Selector  NumberOfDimensions=2  InputPortWidth=ROBOT_DOF  IndexOptions=Index vector (dialog),Index vector (dialog)  Indices=[1:ROBOT_DOF],1  OutputSizes=1,1
  Selector4 : Selector  NumberOfDimensions=2  InputPortWidth=3  IndexOptions=Index vector (dialog),Index vector (dialog)  Indices=[1:3],[1:3]  OutputSizes=1,1
  Selector6 : Selector  NumberOfDimensions=2  InputPortWidth=3  IndexOptions=Index vector (dialog),Index vector (dialog)  Indices=[1:3],1  OutputSizes=1,1
  Selector7 : Selector  NumberOfDimensions=2  InputPortWidth=ROBOT_DOF  IndexOptions=Index vector (dialog),Index vector (dialog)  Indices=[1:ROBOT_DOF],1  OutputSizes=1,1
  Selector8 : Selector  NumberOfDimensions=2  InputPortWidth=3  IndexOptions=Index vector (dialog),Index vector (dialog)  Indices=[4:6],[1:3]  OutputSizes=1,1
  Selector9 : Selector  NumberOfDimensions=2  InputPortWidth=3  IndexOptions=Index vector (dialog),Index vector (dialog)  Indices=[4:6],[1:3]  OutputSizes=1,1
  Smooth Reference Orientations : Subsystem
  Smooth Reference Positions : Subsystem
  pos_vel_acc_CoM_des : Outport
  pose_vel_acc_LFoot_des : Outport  Port=2
  pose_vel_acc_RFoot_des : Outport  Port=3
  orient_vel_acc_rot_task_des : Outport  Port=4
  s_sDot_sDDot_ref : Outport  Port=5
  tag scope: s_des=global
  wires:
  references_CoM/1 -> Choose Smoothed or Direct References/5(references_CoM), Selector1/1
  Selector1/1 -> Smooth Reference Positions/1(pos_CoM_des)
  references_LFoot/1 -> Choose Smoothed or Direct References/6(references_LFoot), Selector9/1, Selector2/1
  Selector2/1 -> Smooth Reference Positions/2(pos_LFoot_des)
  references_RFoot/1 -> Selector8/1, Choose Smoothed or Direct References/7(references_RFoot), Selector6/1
  Selector6/1 -> Smooth Reference Positions/3(pos_RFoot_des)
  references_s/1 -> Choose Smoothed or Direct References/8(references_s), Selector7/1
  Selector7/1 -> Smooth Reference Positions/4(s_des)
  references_rot_task/1 -> Choose Smoothed or Direct References/9(references_rot_task), Selector4/1
  Selector4/1 -> Smooth Reference Orientations/3(w_R_Rot_task_des)
  Selector8/1 -> Smooth Reference Orientations/2(w_R_RFoot_des)
  Selector9/1 -> Smooth Reference Orientations/1(w_R_LFoot_des)
  Smooth Reference Positions/1(smooth_references_CoM) -> Choose Smoothed or Direct References/1(smooth_references_CoM)
  Smooth Reference Orientations/3(smooth_orient_vel_acc_Rot_task) -> Choose Smoothed or Direct References/12(smooth_references_rot_task)
  Smooth Reference Orientations/2(smooth_orient_vel_acc_RFoot) -> Choose Smoothed or Direct References/11(smooth_orient_vel_acc_RFoot)
  Smooth Reference Orientations/1(smooth_orient_vel_acc_LFoot) -> Choose Smoothed or Direct References/10(smooth_orient_vel_acc_LFoot)
  Choose Smoothed or Direct References/1(pos_vel_acc_CoM_des) -> pos_vel_acc_CoM_des/1
  Choose Smoothed or Direct References/2(pose_vel_acc_LFoot_des) -> pose_vel_acc_LFoot_des/1
  Choose Smoothed or Direct References/4(orient_vel_acc_rot_task_des) -> orient_vel_acc_rot_task_des/1
  Choose Smoothed or Direct References/3(pose_vel_acc_RFoot_des) -> pose_vel_acc_RFoot_des/1
  state/1 -> Smooth Reference Positions/5(state), Smooth Reference Orientations/4(state)
  Smooth Reference Positions/2(smooth_pos_vel_acc_LFoot) -> Choose Smoothed or Direct References/2(smooth_pos_vel_acc_LFoot)
  Smooth Reference Positions/3(smooth_pos_vel_acc_RFoot) -> Choose Smoothed or Direct References/3(smooth_pos_vel_acc_RFoot)
  Smooth Reference Positions/4(smooth_references_s) -> Choose Smoothed or Direct References/4(smooth_references_s)
  Choose Smoothed or Direct References/5(s_sDot_sDDot_ref) -> Selector3/1, s_sDot_sDDot_ref/1
  Selector3/1 -> [s_des]

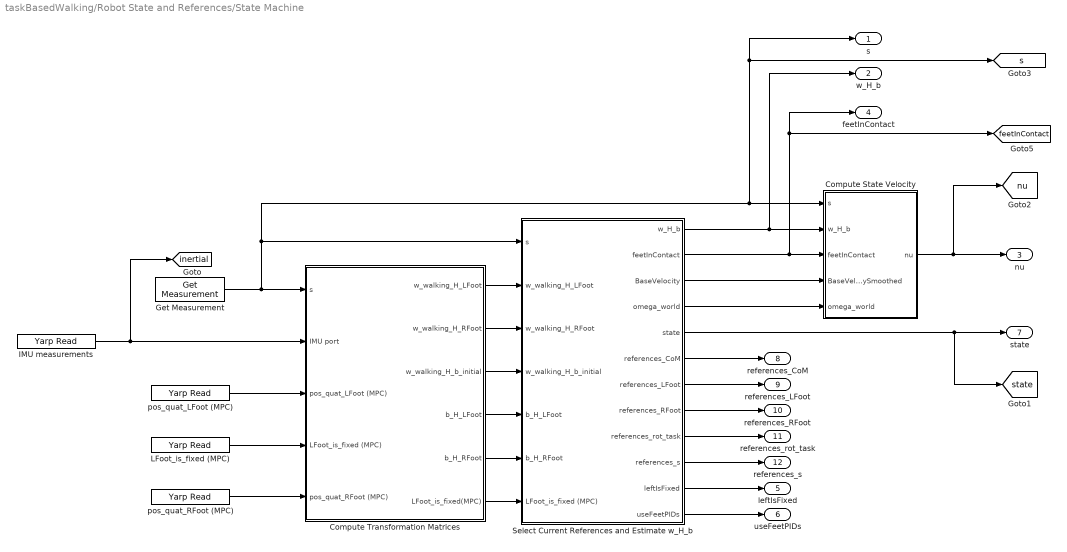
== system taskBasedWalking/Robot State and References/State Machine ==
  Compute State Velocity : Subsystem
  Compute Transformation Matrices : Subsystem
  Get Measurement : WBToolboxLibrary/wholeBodyStates/Get Measurement  measuredType=Joints Position
  IMU measurements : WBToolboxLibrary/Utilities/Yarp Read  portName=Ports.IMU  signalSize=12  timeout=0.5  blocking=off  timestamp=off  autoconnect=on  errorOnConnection=off
  LFoot_is_fixed (MPC) : WBToolboxLibrary/Utilities/Yarp Read  portName=Ports.LFOOT_IS_FIXED  signalSize=1  timeout=0.5  blocking=off  timestamp=off  autoconnect=on  errorOnConnection=off
  Select Current References and Estimate w_H_b : Subsystem
  pos_quat_LFoot (MPC) : WBToolboxLibrary/Utilities/Yarp Read  portName=Ports.LFOOT_DES  signalSize=7  timeout=0.5  blocking=off  timestamp=off  autoconnect=on  errorOnConnection=off
  "pos_quat_RFoot (MPC) " : WBToolboxLibrary/Utilities/Yarp Read  portName=Ports.RFOOT_DES  signalSize=7  timeout=0.5  blocking=off  timestamp=off  autoconnect=on  errorOnConnection=off
  s : Outport
  w_H_b : Outport  Port=2
  nu : Outport  Port=3
  feetInContact : Outport  Port=4
  leftIsFixed : Outport  Port=5
  useFeetPIDs : Outport  Port=6
  state : Outport  Port=7
  references_CoM : Outport  Port=8
  references_LFoot : Outport  Port=9
  references_RFoot : Outport  Port=10
  references_rot_task : Outport  Port=11
  references_s : Outport  Port=12
  tag scope: feetInContact=global, inertial=global, nu=global, s=global, state=global
  wires:
  Get Measurement/1 -> s/1, [s], Compute State Velocity/1(s), Select Current References and Estimate w_H_b/1(s), Compute Transformation Matrices/1(s)
  IMU measurements/1 -> [inertial], Compute Transformation Matrices/2(IMU port)
  pos_quat_LFoot (MPC)/1 -> Compute Transformation Matrices/3(pos_quat_LFoot (MPC))
  "pos_quat_RFoot (MPC) "/1 -> Compute Transformation Matrices/5("pos_quat_RFoot (MPC) ")
  Compute Transformation Matrices/1(w_walking_H_LFoot) -> Select Current References and Estimate w_H_b/2(w_walking_H_LFoot)
  Compute Transformation Matrices/2(w_walking_H_RFoot) -> Select Current References and Estimate w_H_b/3(w_walking_H_RFoot)
  Compute Transformation Matrices/3(w_walking_H_b_initial) -> Select Current References and Estimate w_H_b/4(w_walking_H_b_initial)
  Select Current References and Estimate w_H_b/1(w_H_b) -> Compute State Velocity/2(w_H_b), w_H_b/1
  Select Current References and Estimate w_H_b/2(feetInContact) -> feetInContact/1, [feetInContact], Compute State Velocity/3("feetInContact ")
  Compute State Velocity/1(nu) -> [nu], nu/1
  Select Current References and Estimate w_H_b/5(state) -> state/1, [state]
  Select Current References and Estimate w_H_b/10(references_s) -> references_s/1
  Select Current References and Estimate w_H_b/6(references_CoM) -> references_CoM/1
  Select Current References and Estimate w_H_b/9(references_rot_task) -> references_rot_task/1
  Select Current References and Estimate w_H_b/8(references_RFoot) -> references_RFoot/1
  Select Current References and Estimate w_H_b/7(references_LFoot) -> references_LFoot/1
  Compute Transformation Matrices/4("b_H_LFoot ") -> Select Current References and Estimate w_H_b/5(b_H_LFoot)
  Compute Transformation Matrices/5(b_H_RFoot) -> Select Current References and Estimate w_H_b/6(b_H_RFoot)
  LFoot_is_fixed (MPC)/1 -> Compute Transformation Matrices/4(LFoot_is_fixed (MPC))
  Compute Transformation Matrices/6(LFoot_is_fixed(MPC)) -> Select Current References and Estimate w_H_b/7(LFoot_is_fixed (MPC))
  Select Current References and Estimate w_H_b/11(leftIsFixed) -> leftIsFixed/1
  Select Current References and Estimate w_H_b/12(useFeetPIDs) -> useFeetPIDs/1
  Select Current References and Estimate w_H_b/3(BaseVelocity) -> Compute State Velocity/4(BaseVelocitySmoothed)
  Select Current References and Estimate w_H_b/4("omega_world ") -> Compute State Velocity/5(omega_world)

== system taskBasedWalking/Robot State and References/emergency stop: joint limits ==
  s   EMERGENCY STOP : Inport
  Enable : EnablePort
  Assertion : Assertion
  Get Limits : WBToolboxLibrary/wholeBodyStates/Get Limits  limitsSource=ControlBoard  limitsType=Position
  MATLAB Function : MATLAB Function  TreatAsAtomicUnit=on
  index1 : Constant  Value=0.01  VectorParams1D=off
  wires:
  Get Limits/1 -> MATLAB Function/1(umin)
  Get Limits/2 -> MATLAB Function/2(umax)
  index1/1 -> MATLAB Function/4(tol)
  s   EMERGENCY STOP/1 -> MATLAB Function/3(u)
  MATLAB Function/1(inRange) -> Assertion/1

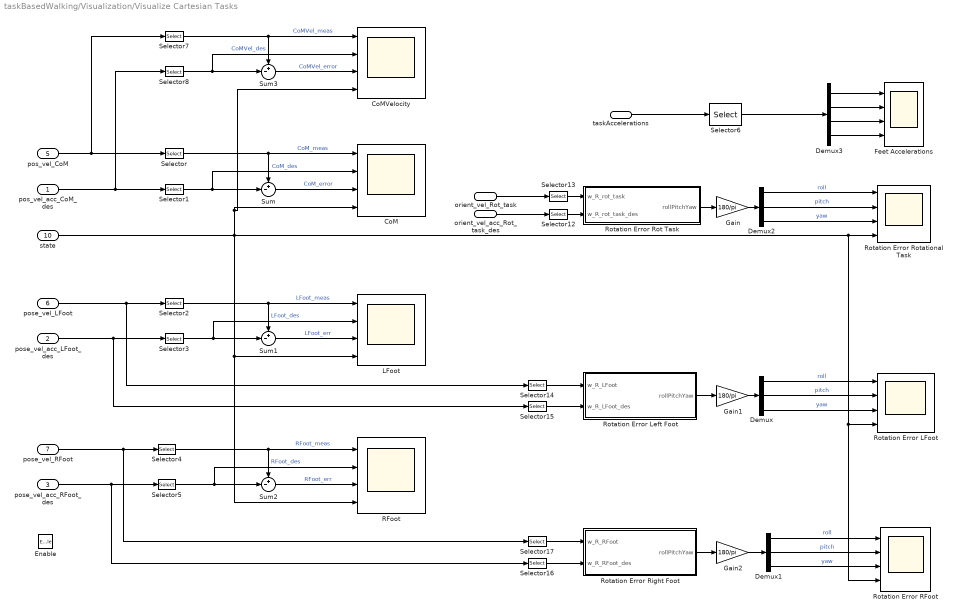
== system taskBasedWalking/Visualization/Visualize Cartesian Tasks ==
  pos_vel_acc_CoM_des : Inport
  pose_vel_acc_LFoot_des : Inport  Port=2
  pose_vel_acc_RFoot_des : Inport  Port=3
  orient_vel_acc_Rot_task_des : Inport  Port=4
  pos_vel_CoM : Inport  Port=5
  pose_vel_LFoot : Inport  Port=6
  pose_vel_RFoot : Inport  Port=7
  orient_vel_Rot_task : Inport  Port=8
  taskAccelerations : Inport  Port=9
  state : Inport  Port=10
  Enable : EnablePort
  CoM : Scope  NumInputPorts=4
  CoMVelocity : Scope  NumInputPorts=4
  Demux : Demux  Outputs=3
  Demux1 : Demux  Outputs=3
  Demux2 : Demux  Outputs=3
  Demux3 : Demux  Outputs=[3;3;3;3]
  Feet Accelerations : Scope  NumInputPorts=4
  Gain : Gain  Gain=180/pi
  Gain1 : Gain  Gain=180/pi
  Gain2 : Gain  Gain=180/pi
  LFoot : Scope  NumInputPorts=4
  RFoot : Scope  NumInputPorts=4
  Rotation Error LFoot : Scope  NumInputPorts=4
  Rotation Error Left Foot : Subsystem
  Rotation Error RFoot : Scope  NumInputPorts=4
  Rotation Error Right Foot : Subsystem
  Rotation Error Rot Task : Subsystem
  Rotation Error Rotational Task : Scope  NumInputPorts=4
  Selector{,1..5} (6 alike) : Selector  NumberOfDimensions=2  InputPortWidth=3  IndexOptions=Index vector (dialog),Index vector (dialog)  Indices=[1:3],1  OutputSizes=1,1
  Selector12 : Selector  NumberOfDimensions=2  InputPortWidth=3  IndexOptions=Index vector (dialog),Index vector (dialog)  Indices=[1:3],[1:3]  OutputSizes=1,1
  Selector13 : Selector  NumberOfDimensions=2  InputPortWidth=3  IndexOptions=Index vector (dialog),Index vector (dialog)  Indices=[1:3],[1:3]  OutputSizes=1,1
  Selector{14..17} (4 alike) : Selector  NumberOfDimensions=2  InputPortWidth=3  IndexOptions=Index vector (dialog),Index vector (dialog)  Indices=[4:6],[1:3]  OutputSizes=1,1
  Selector6 : Selector  InputPortWidth=18  IndexOptions=Index vector (dialog)  Indices=[1:12]  OutputSizes=1
  Selector7 : Selector  NumberOfDimensions=2  InputPortWidth=3  IndexOptions=Index vector (dialog),Index vector (dialog)  Indices=[1:3],2  OutputSizes=1,1
  Selector8 : Selector  NumberOfDimensions=2  InputPortWidth=3  IndexOptions=Index vector (dialog),Index vector (dialog)  Indices=[1:3],2  OutputSizes=1,1
  Sum{,1..3} (4 alike) : Sum  Inputs=+-|
  wires:
  Selector1/1 -> CoM/2, Sum/2  "CoM_des"
  Selector2/1 -> Sum1/1, LFoot/1  "LFoot_meas"
  Selector3/1 -> Sum1/2, LFoot/2  "LFoot_des"
  Selector4/1 -> Sum2/1, RFoot/1  "RFoot_meas"
  Selector5/1 -> RFoot/2, Sum2/2  "RFoot_des"
  pose_vel_RFoot/1 -> Selector4/1, Selector17/1
  pose_vel_acc_RFoot_des/1 -> Selector5/1, Selector16/1
  pose_vel_LFoot/1 -> Selector2/1, Selector14/1
  pose_vel_acc_LFoot_des/1 -> Selector15/1, Selector3/1
  orient_vel_acc_Rot_task_des/1 -> Selector12/1
  orient_vel_Rot_task/1 -> Selector13/1
  Selector/1 -> Sum/1, CoM/1  "CoM_meas"
  Sum/1 -> CoM/3  "CoM_error"
  Sum1/1 -> LFoot/3  "LFoot_err"
  Sum2/1 -> RFoot/3  "RFoot_err"
  Selector14/1 -> Rotation Error Left Foot/1(w_R_LFoot)
  Selector15/1 -> Rotation Error Left Foot/2(w_R_LFoot_des)
  Rotation Error Left Foot/1(rollPitchYaw) -> Gain1/1
  Demux/1 -> Rotation Error LFoot/1  "roll"
  Demux/2 -> Rotation Error LFoot/2  "pitch"
  Demux/3 -> Rotation Error LFoot/3  "yaw"
  Selector17/1 -> Rotation Error Right Foot/1(w_R_RFoot)
  Selector16/1 -> Rotation Error Right Foot/2(w_R_RFoot_des)
  Rotation Error Right Foot/1(rollPitchYaw) -> Gain2/1
  Demux1/1 -> Rotation Error RFoot/1  "roll"
  Demux1/2 -> Rotation Error RFoot/2  "pitch"
  Demux1/3 -> Rotation Error RFoot/3  "yaw"
  Selector13/1 -> Rotation Error Rot Task/1(w_R_rot_task)
  Selector12/1 -> Rotation Error Rot Task/2(w_R_rot_task_des)
  Rotation Error Rot Task/1(rollPitchYaw) -> Gain/1
  Demux2/1 -> Rotation Error Rotational Task/1  "roll"
  Demux2/2 -> Rotation Error Rotational Task/2  "pitch"
  Demux2/3 -> Rotation Error Rotational Task/3  "yaw"
  Gain/1 -> Demux2/1
  Gain1/1 -> Demux/1
  Gain2/1 -> Demux1/1
  Selector6/1 -> Demux3/1
  Demux3/2 -> Feet Accelerations/2
  Demux3/1 -> Feet Accelerations/1
  taskAccelerations/1 -> Selector6/1
  Demux3/3 -> Feet Accelerations/3
  Demux3/4 -> Feet Accelerations/4
  Sum3/1 -> CoMVelocity/3  "CoMVel_error"
  Selector7/1 -> CoMVelocity/1, Sum3/1  "CoMVel_meas"
  state/1 -> Rotation Error Rotational Task/4, Rotation Error LFoot/4, Rotation Error RFoot/4, CoMVelocity/4, CoM/4, RFoot/4, LFoot/4
  pos_vel_acc_CoM_des/1 -> Selector8/1, Selector1/1
  pos_vel_CoM/1 -> Selector7/1, Selector/1
  Selector8/1 -> Sum3/2, CoMVelocity/2  "CoMVel_des"

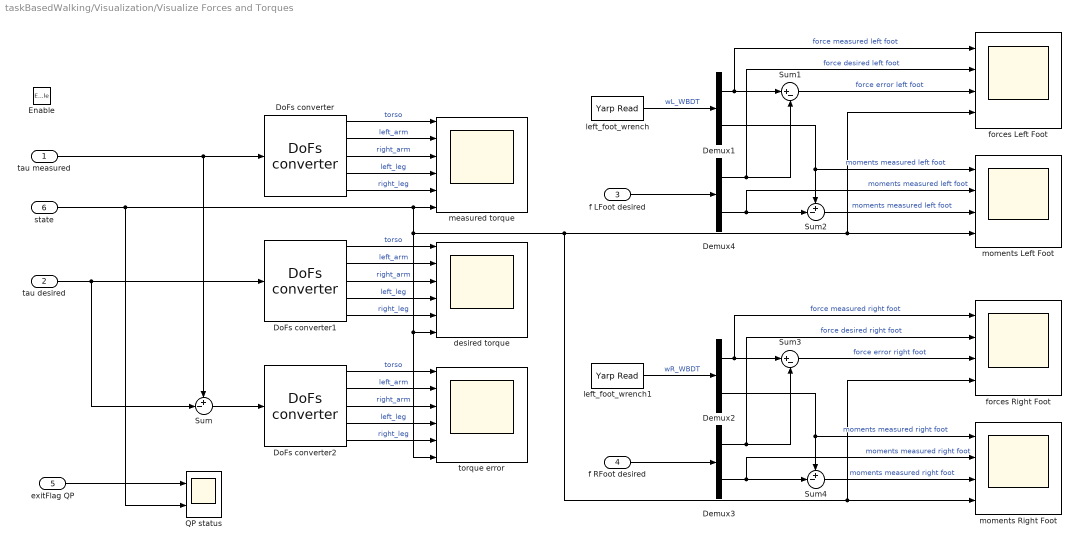
== system taskBasedWalking/Visualization/Visualize Forces and Torques ==
  tau measured : Inport
  tau desired : Inport  Port=2
  f LFoot desired : Inport  Port=3
  f RFoot desired : Inport  Port=4
  exitFlag QP : Inport  Port=5
  state : Inport  Port=6
  Enable : EnablePort
  Demux{1..4} (4 alike) : Demux  Outputs=[3;3]
  DoFs converter : WBToolboxLibrary/Utilities/DoFs converter  yarp2WBIOption=From YARP to WBI
  DoFs converter1 : WBToolboxLibrary/Utilities/DoFs converter  yarp2WBIOption=From YARP to WBI
  DoFs converter2 : WBToolboxLibrary/Utilities/DoFs converter  yarp2WBIOption=From YARP to WBI
  QP status : Scope  NumInputPorts=2
  Sum : Sum  Inputs=+-|
  Sum1 : Sum  Inputs=|+-
  Sum2 : Sum  Inputs=+-|
  Sum3 : Sum  Inputs=|+-
  Sum4 : Sum  Inputs=+-|
  desired torque : Scope  NumInputPorts=6
  forces Left Foot : Scope  NumInputPorts=4
  forces Right Foot : Scope  NumInputPorts=4
  left_foot_wrench : WBToolboxLibrary/Utilities/Yarp Read  portName=Ports.LEFT_FOOT_EXT_WRENCH  signalSize=6  timeout=0.5  blocking=off  timestamp=off  autoconnect=on  errorOnConnection=on
  left_foot_wrench1 : WBToolboxLibrary/Utilities/Yarp Read  portName=Ports.RIGHT_FOOT_EXT_WRENCH  signalSize=6  timeout=0.5  blocking=off  timestamp=off  autoconnect=on  errorOnConnection=on
  measured torque : Scope  NumInputPorts=6
  moments Left Foot : Scope  NumInputPorts=4
  moments Right Foot : Scope  NumInputPorts=4
  torque error : Scope  NumInputPorts=6
  wires:
  Sum2/1 -> moments Left Foot/3  "moments measured left foot"
  state/1 -> QP status/2, torque error/6, desired torque/6, forces Right Foot/4, moments Right Foot/4, forces Left Foot/4, moments Left Foot/4, measured torque/6
  DoFs converter1/2 -> desired torque/2  "left_arm"
  Demux4/1 -> forces Left Foot/2, Sum1/2  "force desired left foot"
  DoFs converter2/1 -> torque error/1  "torso"
  DoFs converter1/4 -> desired torque/4  "left_leg"
  Demux4/2 -> moments Left Foot/2, Sum2/2  "moments measured left foot"
  DoFs converter/1 -> measured torque/1  "torso"
  DoFs converter2/3 -> torque error/3  "right_arm"
  f RFoot desired/1 -> Demux3/1
  DoFs converter1/1 -> desired torque/1  "torso"
  Sum4/1 -> moments Right Foot/3  "moments measured right foot"
  tau desired/1 -> Sum/2, DoFs converter1/1
  Demux2/1 -> forces Right Foot/1, Sum3/1  "force measured right foot"
  DoFs converter2/2 -> torque error/2  "left_arm"
  Sum3/1 -> forces Right Foot/3  "force error right foot"
  DoFs converter/5 -> measured torque/5  "right_leg"
  DoFs converter2/5 -> torque error/5  "right_leg"
  exitFlag QP/1 -> QP status/1
  left_foot_wrench/1 -> Demux1/1  "wL_WBDT"
  DoFs converter1/3 -> desired torque/3  "right_arm"
  Demux3/1 -> forces Right Foot/2, Sum3/2  "force desired right foot"
  f LFoot desired/1 -> Demux4/1
  Sum1/1 -> forces Left Foot/3  "force error left foot"
  tau measured/1 -> Sum/1, DoFs converter/1
  DoFs converter1/5 -> desired torque/5  "right_leg"
  DoFs converter/2 -> measured torque/2  "left_arm"
  DoFs converter/3 -> measured torque/3  "right_arm"
  Demux3/2 -> moments Right Foot/2, Sum4/2  "moments measured right foot"
  Sum/1 -> DoFs converter2/1
  Demux1/1 -> forces Left Foot/1, Sum1/1  "force measured left foot"
  DoFs converter/4 -> measured torque/4  "left_leg"
  Demux1/2 -> moments Left Foot/1, Sum2/1  "moments measured left foot"
  left_foot_wrench1/1 -> Demux2/1  "wR_WBDT"
  DoFs converter2/4 -> torque error/4  "left_leg"
  Demux2/2 -> moments Right Foot/1, Sum4/1  "moments measured right foot"

== system taskBasedWalking/Visualization/Visualize Gain Scheduling ==
  Kp_CoM : Inport
  Kd_CoM : Inport  Port=2
  Kp_LFoot : Inport  Port=3
  Kd_LFoot : Inport  Port=4
  Kp_RFoot : Inport  Port=5
  Kd_RFoot : Inport  Port=6
  Kp_rot_task : Inport  Port=7
  Kd_rot_task : Inport  Port=8
  impedances : Inport  Port=9
  dampings : Inport  Port=10
  state : Inport  Port=11
  Enable : EnablePort
  DoFs converter1 : WBToolboxLibrary/Utilities/DoFs converter  yarp2WBIOption=From YARP to WBI
  DoFs converter4 : WBToolboxLibrary/Utilities/DoFs converter  yarp2WBIOption=From YARP to WBI
  joint position gains : Scope  NumInputPorts=6
  joint velocity gains : Scope  NumInputPorts=6
  orient gains rot task : Scope  NumInputPorts=2
  pos gains CoM : Scope  NumInputPorts=2
  pose gains LFoot : Scope  NumInputPorts=2
  pose gains RFoot : Scope  NumInputPorts=2
  vel gains CoM : Scope  NumInputPorts=2
  vel gains LFoot : Scope  NumInputPorts=2
  vel gains RFoot : Scope  NumInputPorts=2
  vel gains rot task : Scope  NumInputPorts=2
  wires:
  Kp_CoM/1 -> pos gains CoM/1
  Kp_LFoot/1 -> pose gains LFoot/1
  Kp_RFoot/1 -> pose gains RFoot/1
  Kp_rot_task/1 -> orient gains rot task/1
  state/1 -> vel gains LFoot/2, pose gains LFoot/2, vel gains CoM/2, vel gains rot task/2, orient gains rot task/2, vel gains RFoot/2, joint velocity gains/6, joint position gains/6, pose gains RFoot/2, pos gains CoM/2
  Kd_CoM/1 -> vel gains CoM/1
  Kd_LFoot/1 -> vel gains LFoot/1
  Kd_RFoot/1 -> vel gains RFoot/1
  Kd_rot_task/1 -> vel gains rot task/1
  DoFs converter4/2 -> joint position gains/2  "left_arm"
  DoFs converter4/1 -> joint position gains/1  "torso"
  DoFs converter4/4 -> joint position gains/4  "left_leg"
  DoFs converter4/3 -> joint position gains/3  "right_arm"
  DoFs converter4/5 -> joint position gains/5  "right_leg"
  DoFs converter1/2 -> joint velocity gains/2  "left_arm"
  DoFs converter1/1 -> joint velocity gains/1  "torso"
  DoFs converter1/4 -> joint velocity gains/4  "left_leg"
  DoFs converter1/3 -> joint velocity gains/3  "right_arm"
  DoFs converter1/5 -> joint velocity gains/5  "right_leg"
  impedances/1 -> DoFs converter4/1
  dampings/1 -> DoFs converter1/1
